simulink library "teme_2_eci_lib"  (R2016b)
settings: Solver=ode45  StartTime=0.0  StopTime=10.0  RelTol=1e-3  EnableMultiTasking=on
settings Model: Creator=Taylor  LastModifiedBy=taylorreynolds
settings DataIOCC: LimitDataPoints=on
settings OptimizationCC: LifeSpan=inf
settings DebuggingCC: AllowSymbolicDim=off  SFUnexpectedBacktrackingDiag=warning  SFNoUnconditionalDefaultTransitionDiag=warning  SFExecutionAtInitializationDiag=none
settings GRTTargetCC: TargetLangStandard=C89/C90 (ANSI)  GeneratePreprocessorConditionals=Disable all
settings ConfigComp: CovMetricSettings=dw  CovHtmlReporting=on  CovSaveCumulativeToWorkspaceVar=on  CovSaveSingleToWorkspaceVar=on  CovExternalEMLEnable=off

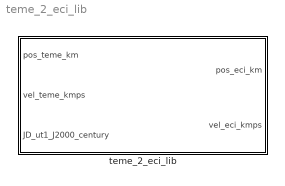
== system teme_2_eci_lib ==
  teme_2_eci_lib : Subsystem

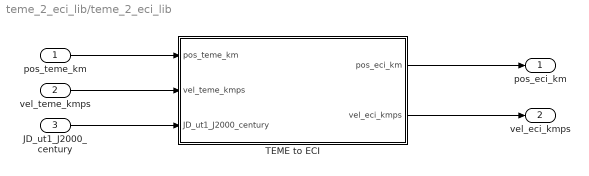
== system teme_2_eci_lib/teme_2_eci_lib ==
  pos_teme_km : Inport
  vel_teme_kmps : Inport  Port=2
  JD_ut1_J2000_century : Inport  Port=3
  TEME to ECI : MATLAB Function  TreatAsAtomicUnit=on
  pos_eci_km : Outport
  vel_eci_kmps : Outport  Port=2
  wires:
  TEME to ECI/2(vel_eci_kmps) -> vel_eci_kmps/1
  JD_ut1_J2000_century/1 -> TEME to ECI/3(JD_ut1_J2000_century)
  vel_teme_kmps/1 -> TEME to ECI/2(vel_teme_kmps)
  pos_teme_km/1 -> TEME to ECI/1(pos_teme_km)
  TEME to ECI/1(pos_eci_km) -> pos_eci_km/1

== matlab function teme_2_eci_lib/TEME to ECI ==
  data: pos_teme_km input; pos_eci_km output; vel_teme_kmps input; JD_ut1_J2000_century input; vel_eci_kmps output
% TEME to ECI ROTATION TRANSFORMATION
%   UW DubSat-1
%   T. Reynolds: 5/14/17
%
%  Transforms a vector from the true equator mean equinox system,
%    (TEME) to the ECI (j2000) system.
%
%  Inputs          
%    - rteme : position in TEME [km]
%    - vteme : velocity in TEME [km/s]
%    - ttt   : Julian centuries of ut1 (approximating TT) [centuries]
%
%  Outputs 
%    - reci  : position vector in ECI [km]
%    - veci  : velocity vector in ECI [km/s]
%
%  References    :
%    Vallado       2013, Ch. 3
% ----------------------------------------------------------------------------

function [pos_eci_km,vel_eci_kmps] = teme2eci  ( pos_teme_km,vel_teme_kmps,JD_ut1_J2000_century )

        prec = precess ( JD_ut1_J2000_century );

        nutteme = truemean ( JD_ut1_J2000_century );

        pos_eci_km = prec * nutteme * pos_teme_km;

        vel_eci_kmps = prec * nutteme * vel_teme_kmps;
end

function prec = precess ( ttt )
        
        convrt = pi / (180.0 * 3600.0);
        ttt2 =  ttt * ttt;
        ttt3 =  ttt2 * ttt;

        zeta =             2306.2181*ttt + 0.30188*ttt2 + 0.017998*ttt3; % "
        theta=             2004.3109*ttt - 0.42665*ttt2 - 0.041833*ttt3;
        z    =             2306.2181*ttt + 1.09468*ttt2 + 0.018203*ttt3;       
        % convert units to rad
        zeta = zeta  * convrt; 
        theta= theta * convrt;
        z    = z     * convrt;

        coszeta  = cos(zeta);
        sinzeta  = sin(zeta);
        costheta = cos(theta);
        sintheta = sin(theta);
        cosz     = cos(z);
        sinz     = sin(z);

        prec=zeros(3);
        % ----------------- form matrix  mod to j2000 -----------------
        prec(1,1) =  coszeta * costheta * cosz - sinzeta * sinz;
        prec(1,2) =  coszeta * costheta * sinz + sinzeta * cosz;
        prec(1,3) =  coszeta * sintheta;
        prec(2,1) = -sinzeta * costheta * cosz - coszeta * sinz;
        prec(2,2) = -sinzeta * costheta * sinz + coszeta * cosz;
        prec(2,3) = -sinzeta * sintheta;
        prec(3,1) = -sintheta * cosz;
        prec(3,2) = -sintheta * sinz;
        prec(3,3) =  costheta;
        
end % precess

function DCMx   = rotxmat( x_ang )
    sx = sin(x_ang);
    cx = cos(x_ang);

    
    DCMx    = [ 1   0   0;
                0   cx  -sx;
                0   sx  cx ];
end

function DCMz   = rotzmat( z_ang )
    sz   = sin(z_ang);
    cz   = cos(z_ang);
    
    DCMz    = [ cz  -sz     0;
                sz  cz      0;
                0   0       1 ];
end

function nutteme = truemean ( ttt )

        DEG2RAD = pi/180.0;
        CONVRT  = 0.0001 * pi / (180*3600.0); % 0.0001" to rad        
        
        % Load nutation parameters
        iau80in_trunc = [ ...
        0  0  0  0  1 -171996   -174.2   92025    8.9    1;
        0  0  2 -2  2  -13187     -1.6    5736   -3.1    9;
        0  0  2  0  2   -2274     -0.2     977   -0.5   31;
        0  0  0  0  2    2062      0.2    -895    0.5    2;
        0  1  0  0  0    1426     -3.4      54   -0.1   10;
        1  0  0  0  0     712      0.1      -7    0     32;
        0  1  2 -2  2    -517      1.2     224   -0.6   11;
        0  0  2  0  1    -386     -0.4     200    0     33;
        1  0  2  0  2    -301      0       129   -0.1   34;
        0 -1  2 -2  2     217     -0.5     -95    0.3   12;
        1  0  0 -2  0    -158      0        -1    0     35;
        0  0  2 -2  1     129      0.1     -70    0     13;
       -1  0  2  0  2     123      0       -53    0     36;
        1  0  0  0  1      63      0.1     -33    0     38;
        0  0  0  2  0      63      0        -2    0     37;
       -1  0  2  2  2     -59      0        26    0     40;
       -1  0  0  0  1     -58     -0.1      32    0     39;
        1  0  2  0  1     -51      0        27    0     41;
        2  0  0 -2  0      48      0         1    0     14;
       -2  0  2  0  1      46      0       -24    0      3;
        0  0  2  2  2     -38      0        16    0     42;
        2  0  2  0  2     -31      0        13    0     45;
        2  0  0  0  0      29      0        -1    0     43;
        1  0  2 -2  2      29      0       -12    0     44;
        0  0  2  0  0      26      0        -1    0     46;
        0  0  2 -2  0     -22      0         0    0     15;
       -1  0  2  0  1      21      0       -10    0     47;
        0  2  0  0  0      17     -0.1       0    0     16;
        0  2  2 -2  2     -16      0.1       7    0     18;
       -1  0  0  2  1      16      0        -8    0     48;
        0  1  0  0  1     -15      0         9    0     17;
        1  0  0 -2  1     -13      0         7    0     49;
        0 -1  0  0  1     -12      0         6    0     19;
        2  0 -2  0  0      11      0         0    0      4;
       -1  0  2  2  1     -10      0         5    0     50;
        1  0  2  2  2      -8      0         3    0     54 ];
    
        iar80   = iau80in_trunc(:,1:5);
        rar80   = iau80in_trunc(:,6:9);
        
       for i=1:36
           for j=1:4
               rar80(i,j)= rar80(i,j) * CONVRT;
           end
       end
        
        % ---- determine coefficients for iau 1980 nutation theory ----
        ttt2= ttt*ttt;
        ttt3= ttt2*ttt;
        ttt4= ttt2*ttt2;

        meaneps = -46.8150 *ttt - 0.00059 *ttt2 + 0.001813 *ttt3 + 84381.448;
        meaneps = rem( meaneps/3600.0 ,360.0  );
        meaneps = meaneps * DEG2RAD;

        l    =  134.96340251  + ( 1717915923.2178 *ttt + ...
                31.8792 *ttt2 + 0.051635 *ttt3 - 0.00024470 *ttt4 ) / 3600.0;
        l1   =  357.52910918  + (  129596581.0481 *ttt - ...
                 0.5532 *ttt2 - 0.000136 *ttt3 - 0.00001149*ttt4 )  / 3600.0;
        f    =   93.27209062  + ( 1739527262.8478 *ttt - ...
                12.7512 *ttt2 + 0.001037 *ttt3 + 0.00000417*ttt4 )  / 3600.0;
        d    =  297.85019547  + ( 1602961601.2090 *ttt - ...
                 6.3706 *ttt2 + 0.006593 *ttt3 - 0.00003169*ttt4 )  / 3600.0;
        omega=  125.04455501  + (   -6962890.2665 *ttt + ...
                 7.4722 *ttt2 + 0.007702 *ttt3 - 0.00005939*ttt4 )  / 3600.0;

        l    = rem( l,360.0  )     * DEG2RAD;
        l1   = rem( l1,360.0  )    * DEG2RAD;
        f    = rem( f,360.0  )     * DEG2RAD;
        d    = rem( d,360.0  )     * DEG2RAD;
        omega= rem( omega,360.0  ) * DEG2RAD;

        deltapsi= 0.0;
        deltaeps= 0.0;

        for i= 1:36   % the eqeterms in nut80.dat are already sorted
            tempval= iar80(i,1)*l + iar80(i,2)*l1 + iar80(i,3)*f + ...
                     iar80(i,4)*d + iar80(i,5)*omega;
            deltapsi= deltapsi + (rar80(i,1)+rar80(i,2)*ttt) * sin( tempval );
            deltaeps= deltaeps + (rar80(i,3)+rar80(i,4)*ttt) * cos( tempval );
        end

        % --------------- find nutation parameters --------------------
        deltapsi = rem( deltapsi,360.0  ) * DEG2RAD;
        deltaeps = rem( deltaeps,360.0  ) * DEG2RAD;
        trueeps  = meaneps + deltaeps;
        cospsi  = cos(deltapsi);
        sinpsi  = sin(deltapsi);
        coseps  = cos(meaneps);
        sineps  = sin(meaneps);
        costrueeps = cos(trueeps);
        sintrueeps = sin(trueeps);

     % NOT SURE ABOUT THIS PART - ASSUMING SIMPLEST ONE TO DROP THE INPUT
%         jdttt = ttt*36525.0 + 2451545.0;
%         % small disconnect with ttt instead of ut1
%         if (jdttt > 2450449.5 ) && (eqeterms > 0)
%             eqe = deltapsi* cos(meaneps) ...
%                 + 0.00264*pi /(3600*180)*sin(omega) ...
%                 + 0.000063*pi /(3600*180)*sin(2.0 *omega);
%         else
            eqe = deltapsi* cos(meaneps);
%         end
        
        nut      = zeros(3);
        nut(1,1) =  cospsi;
        nut(1,2) =  costrueeps * sinpsi;
        nut(1,3) =  sintrueeps * sinpsi;
        nut(2,1) = -coseps * sinpsi;
        nut(2,2) =  costrueeps * coseps * cospsi + sintrueeps * sineps;
        nut(2,3) =  sintrueeps * coseps * cospsi - sineps * costrueeps;
        nut(3,1) = -sineps * sinpsi;
        nut(3,2) =  costrueeps * sineps * cospsi - sintrueeps * coseps;
        nut(3,3) =  sintrueeps * sineps * cospsi + costrueeps * coseps;

        st      = zeros(3);
        st(1,1) =  cos(eqe);
        st(1,2) = -sin(eqe);
        st(1,3) =  0.0;
        st(2,1) =  sin(eqe);
        st(2,2) =  cos(eqe);
        st(2,3) =  0.0;
        st(3,1) =  0.0;
        st(3,2) =  0.0;
        st(3,3) =  1.0;

        nutteme = nut*st;
          
end % function
